simulink model "linearni_quad_trajektorie"  (R2020a)
settings: Solver=VariableStepAuto  StartTime=0.0  StopTime=smax/v  RelTol=1e-3
values from neighbouring files (symbols this model uses):
  a1 = 2    [overeniFunkcionality.m]    (also in sampleQnorm.m)
  a2 = 1.5    [overeniFunkcionality.m]    (also in sampleQnorm.m)
  a3 = 0.5    [overeniFunkcionality.m]    (also in sampleQnorm.m)
  r = a1-a2-a3    (= 0)    [overeniFunkcionality.m]    (also in sampleQnorm.m)
  R = a1+a2+a3    (= 4)    [overeniFunkcionality.m]    (also in sampleQnorm.m)
  s = surf(simulation.s_lin.signals.values,fiss,dQ)    [sampleQnorm.m]
  T_1_0 = [cos(theta10), -sin(theta10), 0, a1*cos(theta10) ... (first row only)    [overeniFunkcionality.m]    (also in sampleQnorm.m)
  T_2_1 = [cos(theta20), -sin(theta20), 0, a2*cos(theta20) ... (first row only)    [overeniFunkcionality.m]    (also in sampleQnorm.m)
  T_3_2 = [cos(theta30), -sin(theta30), 0, a3*cos(theta30) ... (first row only)    [overeniFunkcionality.m]    (also in sampleQnorm.m)
  v = 0.5    [overeniFunkcionality.m]    (also in sampleQnorm.m)
undefined symbols (not defined in the file or in its folder): X, Y, Z
libraries: sm_lib x84, nesl_utility x48
(part 3 of 3)

== system linearni_quad_trajektorie/Manipulator4/LINK 1 ==
  note: SUBSYSTEM RAMENE
  T_CG_1_0 : sm_lib/Frames and Transforms/Rigid Transform  TranslationMethod=Cartesian  TranslationStandardOffset=0  TranslationLengthUnit=m  TranslationStandardAxis=+Z  TranslationCartesianOffset=T_1_0(1:3,4)/2  TranslationROffset=0  TranslationROffsetUnits=m  TranslationZOffset=0  TranslationZOffsetUnits=m  TranslationThetaOffset=0  TranslationThetaOffsetUnits=deg  RotationMethod=RotationMatrix  RotationAngleUnits=deg  RotationStandardAxis=+Z  RotationAngle=0.0  RotationArbitraryAxis=[0 0 1]  FollAlignAxisA=+X  BaseAlignAxisA=+Y  FollAlignAxisB=+Y  BaseAlignAxisB=+Z  RotationSequenceAxes=FollowerAxes  RotationSequence=XYX  RotationSequenceAngles=[0 0 0]  RotationSequenceAnglesUnits=deg  RotationMatrix=T_1_0(1:3,1:3)
  Transform prvniho vuci nultymu = T_1_0 : sm_lib/Frames and Transforms/Rigid Transform  TranslationMethod=Cartesian  TranslationStandardOffset=0  TranslationLengthUnit=m  TranslationStandardAxis=+Z  TranslationCartesianOffset=T_1_0(1:3,4)  TranslationROffset=0  TranslationROffsetUnits=m  TranslationZOffset=0  TranslationZOffsetUnits=m  TranslationThetaOffset=0  TranslationThetaOffsetUnits=deg  RotationMethod=RotationMatrix  RotationAngleUnits=deg  RotationStandardAxis=+Z  RotationAngle=0.0  RotationArbitraryAxis=[0 0 1]  FollAlignAxisA=+X  BaseAlignAxisA=+Y  FollAlignAxisB=+Y  BaseAlignAxisB=+Z  RotationSequenceAxes=FollowerAxes  RotationSequence=XYX  RotationSequenceAngles=[0 0 0]  RotationSequenceAnglesUnits=deg  RotationMatrix=T_1_0(1:3,1:3)
  graficky objekt : sm_lib/Body Elements/Brick Solid  GraphicAmbientColor=[0.15 0.15 0.15 1.0]  BasedOnType=Density  BrickDimensions=[a1 0.05 0.05]  BrickDimensionUnits=m  CenterOfMass=[0 0 0]  CenterOfMassUnits=m  GraphicDiffuseColor=[0.5 0.5 0.5]  Density=1000  DensityUnits=kg/m^3  DoExposeReferenceFrame=on  GraphicEmissiveColor=[0.0 0.0 0.0 1.0]  ExportEntireGeometry=off  SerializedFrames=<Frames/>  MarkerShape=Sphere  MarkerSize=10  GraphicType=FromGeometry  InertiaType=CalculateFromGeometry  Mass=1  MassUnits=kg  MomentsOfInertia=[1 1 1]  MomentsOfInertiaUnits=kg*m^2  GraphicOpacity=1.0  ProductsOfInertia=[0 0 0]  ProductsOfInertiaUnits=kg*m^2  GraphicShininess=75  GraphicSpecularColor=[0.5 0.5 0.5 1.0]  GraphicVisPropType=SimpleVisualProperties
  CS_A : PMIOPort  Side=Left
  CS_B : PMIOPort  Port=2  Side=Right
  connections:
  Transform prvniho vuci nultymu = T_1_0/LConn1 -- CS_A/RConn1 -- T_CG_1_0/LConn1
  CS_B/RConn1 -- Transform prvniho vuci nultymu = T_1_0/RConn1
  graficky objekt/RConn1 -- T_CG_1_0/RConn1

== system linearni_quad_trajektorie/Manipulator4/LINK 2 ==
  note: SUBSYSTEM RAMENE
  T_CG_2_1 : sm_lib/Frames and Transforms/Rigid Transform  TranslationMethod=Cartesian  TranslationStandardOffset=0  TranslationLengthUnit=m  TranslationStandardAxis=+Z  TranslationCartesianOffset=T_2_1(1:3,4)/2  TranslationROffset=0  TranslationROffsetUnits=m  TranslationZOffset=0  TranslationZOffsetUnits=m  TranslationThetaOffset=0  TranslationThetaOffsetUnits=deg  RotationMethod=RotationMatrix  RotationAngleUnits=deg  RotationStandardAxis=+Z  RotationAngle=0.0  RotationArbitraryAxis=[0 0 1]  FollAlignAxisA=+X  BaseAlignAxisA=+Y  FollAlignAxisB=+Y  BaseAlignAxisB=+Z  RotationSequenceAxes=FollowerAxes  RotationSequence=XYX  RotationSequenceAngles=[0 0 0]  RotationSequenceAnglesUnits=deg  RotationMatrix=T_2_1(1:3,1:3)
  Transform druhyho vuci prvnimu = T_2_1 : sm_lib/Frames and Transforms/Rigid Transform  TranslationMethod=Cartesian  TranslationStandardOffset=0  TranslationLengthUnit=m  TranslationStandardAxis=+Z  TranslationCartesianOffset=T_2_1(1:3,4)  TranslationROffset=0  TranslationROffsetUnits=m  TranslationZOffset=0  TranslationZOffsetUnits=m  TranslationThetaOffset=0  TranslationThetaOffsetUnits=deg  RotationMethod=RotationMatrix  RotationAngleUnits=deg  RotationStandardAxis=+Z  RotationAngle=0.0  RotationArbitraryAxis=[0 0 1]  FollAlignAxisA=+X  BaseAlignAxisA=+Y  FollAlignAxisB=+Y  BaseAlignAxisB=+Z  RotationSequenceAxes=FollowerAxes  RotationSequence=XYX  RotationSequenceAngles=[0 0 0]  RotationSequenceAnglesUnits=deg  RotationMatrix=T_2_1(1:3,1:3)
  graficky objekt : sm_lib/Body Elements/Brick Solid  GraphicAmbientColor=[0.15 0.15 0.15 1.0]  BasedOnType=Density  BrickDimensions=[a2 0.05 0.05]  BrickDimensionUnits=m  CenterOfMass=[0 0 0]  CenterOfMassUnits=m  GraphicDiffuseColor=[0.5 0.5 0.5]  Density=1000  DensityUnits=kg/m^3  DoExposeReferenceFrame=on  GraphicEmissiveColor=[0.0 0.0 0.0 1.0]  ExportEntireGeometry=off  SerializedFrames=<Frames/>  MarkerShape=Sphere  MarkerSize=10  GraphicType=FromGeometry  InertiaType=CalculateFromGeometry  Mass=1  MassUnits=kg  MomentsOfInertia=[1 1 1]  MomentsOfInertiaUnits=kg*m^2  GraphicOpacity=1.0  ProductsOfInertia=[0 0 0]  ProductsOfInertiaUnits=kg*m^2  GraphicShininess=75  GraphicSpecularColor=[0.5 0.5 0.5 1.0]  GraphicVisPropType=SimpleVisualProperties
  CS_A : PMIOPort  Side=Left
  CS_B : PMIOPort  Port=2  Side=Right
  connections:
  T_CG_2_1/LConn1 -- Transform druhyho vuci prvnimu = T_2_1/LConn1 -- CS_A/RConn1
  CS_B/RConn1 -- Transform druhyho vuci prvnimu = T_2_1/RConn1
  graficky objekt/RConn1 -- T_CG_2_1/RConn1

== system linearni_quad_trajektorie/Manipulator4/LINK 3 ==
  note: SUBSYSTEM RAMENE
  T_CG_3_2 : sm_lib/Frames and Transforms/Rigid Transform  TranslationMethod=Cartesian  TranslationStandardOffset=0  TranslationLengthUnit=m  TranslationStandardAxis=+Z  TranslationCartesianOffset=T_3_2(1:3,4)/2  TranslationROffset=0  TranslationROffsetUnits=m  TranslationZOffset=0  TranslationZOffsetUnits=m  TranslationThetaOffset=0  TranslationThetaOffsetUnits=deg  RotationMethod=RotationMatrix  RotationAngleUnits=deg  RotationStandardAxis=+Z  RotationAngle=0.0  RotationArbitraryAxis=[0 0 1]  FollAlignAxisA=+X  BaseAlignAxisA=+Y  FollAlignAxisB=+Y  BaseAlignAxisB=+Z  RotationSequenceAxes=FollowerAxes  RotationSequence=XYX  RotationSequenceAngles=[0 0 0]  RotationSequenceAnglesUnits=deg  RotationMatrix=T_3_2(1:3,1:3)
  Transform tretiho vuci druhymu = T_3_2 : sm_lib/Frames and Transforms/Rigid Transform  TranslationMethod=Cartesian  TranslationStandardOffset=0  TranslationLengthUnit=m  TranslationStandardAxis=+Z  TranslationCartesianOffset=T_3_2(1:3,4)  TranslationROffset=0  TranslationROffsetUnits=m  TranslationZOffset=0  TranslationZOffsetUnits=m  TranslationThetaOffset=0  TranslationThetaOffsetUnits=deg  RotationMethod=RotationMatrix  RotationAngleUnits=deg  RotationStandardAxis=+Z  RotationAngle=0.0  RotationArbitraryAxis=[0 0 1]  FollAlignAxisA=+X  BaseAlignAxisA=+Y  FollAlignAxisB=+Y  BaseAlignAxisB=+Z  RotationSequenceAxes=FollowerAxes  RotationSequence=XYX  RotationSequenceAngles=[0 0 0]  RotationSequenceAnglesUnits=deg  RotationMatrix=T_3_2(1:3,1:3)
  graficky objekt : sm_lib/Body Elements/Brick Solid  GraphicAmbientColor=[0.15 0.15 0.15 1.0]  BasedOnType=Density  BrickDimensions=[a3 0.05 0.05]  BrickDimensionUnits=m  CenterOfMass=[0 0 0]  CenterOfMassUnits=m  GraphicDiffuseColor=[0.5 0.5 0.5]  Density=1000  DensityUnits=kg/m^3  DoExposeReferenceFrame=on  GraphicEmissiveColor=[0.0 0.0 0.0 1.0]  ExportEntireGeometry=off  SerializedFrames=<Frames/>  MarkerShape=Sphere  MarkerSize=10  GraphicType=FromGeometry  InertiaType=CalculateFromGeometry  Mass=1  MassUnits=kg  MomentsOfInertia=[1 1 1]  MomentsOfInertiaUnits=kg*m^2  GraphicOpacity=1.0  ProductsOfInertia=[0 0 0]  ProductsOfInertiaUnits=kg*m^2  GraphicShininess=75  GraphicSpecularColor=[0.5 0.5 0.5 1.0]  GraphicVisPropType=SimpleVisualProperties
  CS_A : PMIOPort  Side=Left
  CS_B : PMIOPort  Port=2  Side=Right
  connections:
  T_CG_3_2/LConn1 -- Transform tretiho vuci druhymu = T_3_2/LConn1 -- CS_A/RConn1
  CS_B/RConn1 -- Transform tretiho vuci druhymu = T_3_2/RConn1
  graficky objekt/RConn1 -- T_CG_3_2/RConn1

== matlab function linearni_quad_trajektorie/Linearni phi trajektorie1 ==
  data: s input; Xstar output size=3; v input; a input; dXstar output size=3; ddXstar output size=3
function [Xstar, dXstar, ddXstar] = MCSstar(s, v, a)

    A = [2 0.5]';
    B = [0 1]';
%     B = [1 1]';
    C = [2 2.5]';
%     sC = -A;

    r = 0.3;
    vmax = 1;
    
    fi_s = pi/2;
    fi_e = 0;
    
    if v > vmax
        v = vmax;
    else
        v = v;
    end
    nba = (A - B)/norm(A-B);
    nbc = (C-B)/norm(C-B);
    nbs = (nba+nbc)/norm(nba+nbc);
    K1 = (nba*nba'*nbs-nbs);
    l = r/(sqrt(K1'*K1));
    S = B+nbs*l;
    k = nba'*(A-S);
    Pa = A-nba*k;
    Pc = B + norm(Pa-B)*nbc;
    
%     
%     x_pab = A-k1.*nba
    Pb = B;

    helper = (Pa-S);
    fi_pa = atan2(helper(2),helper(1));
    dir = -1;
    deltafi = acos(((Pc-S)'*(Pa-S))/r^2);
    
    s1 = norm(Pa-A);
    s2 = norm(Pc-C);
    sk = r*deltafi;
    smax = s1+s2+sk;
    if s < s1
        k1 = s;
        dk1 = v;
        ddk1 = a;
        Xstar_tmp = A-k1*nba;
        dXstar_tmp = -dk1*nba;
        ddXstar_tmp = -ddk1*nba;
    elseif s1 <= s &&  s < s1+sk
        Phi = (s-s1)/r;
        dPhi = v/r;
        ddPhi = a/r;
        
        Xstar_tmp = r* [cos(fi_pa + dir*Phi); sin(fi_pa + dir*Phi)] + S;
        dXstar_tmp = r* [-sin(fi_pa + dir*Phi); cos(fi_pa + dir*Phi)]*dir*dPhi;
        ddXstar_tmp = r* [-cos(fi_pa + dir*Phi); -sin(fi_pa + dir*Phi)]*dPhi^2 + r* [-sin(fi_pa + dir*Phi); cos(fi_pa + dir*Phi)]*dir*ddPhi;
    elseif s1+sk < s && s < s1+sk+s2
        k2 = s-s1-sk;
        dk2 = v;
        ddk2 = a;
        
        Xstar_tmp = Pc + k2*nbc;
        dXstar_tmp = dk2*nbc;
        ddXstar_tmp = ddk2*nbc;
    else
%         display('ERROR V TRAJEKTORII')
        Xstar_tmp = C;
        dXstar_tmp = zeros(2,1);
        ddXstar_tmp = zeros(2,1);
    end
    
    
    fi = fi_s - fi_s/smax*s;
    dfi = -fi_s/(smax/v);
    ddfi = 0;

    
    Xstar = [Xstar_tmp; fi];
    dXstar = [dXstar_tmp; dfi];
    ddXstar = [ddXstar_tmp; ddfi];
    
end

== matlab function linearni_quad_trajektorie/MATLAB Function2 ==
  data: x input; y input; phi input; dx input; dy input; dphi input; ddx input; ddy input; ddphi input; a1 parameter; a2 parameter; a3 parameter; theta1 output size=1; theta2 output size=1; theta3 output size=1; theta1_dot output size=1; theta2_dot output size=1; theta3_dot output size=1; theta1_dot_dot output size=1; theta2_dot_dot output size=1; theta3_dot_dot output size=1
function [theta1, theta2, theta3,theta1_dot,theta2_dot,theta3_dot,theta1_dot_dot,theta2_dot_dot,theta3_dot_dot] = IOKU( x, y, phi, dx, dy, dphi, ddx, ddy, ddphi, a1, a2, a3)

% theta2
cosQ2 = ((x - a3*cos(phi))^2 + (y - a3*sin(phi))^2 - a1^2 - a2^2)/(2 * a1 * a2);
sinQ2 = -abs(sqrt(abs(1 - cosQ2^2)));
theta2 = atan2(sinQ2, cosQ2);

% theta1
A = [-a2 * sin(theta2), a2 * cos(theta2) + a1; a2 * cos(theta2) + a1, a2 * sin(theta2)];
B = [x - a3*cos(phi); y - a3*sin(phi)];
X = A\B;
theta1 = atan2(X(1), X(2));

% theta3
theta3 = phi - theta1 - theta2;

% uhlova rychlost
JQ = [-a3 * sin(theta1 + theta2 + theta3) - a2 * sin(theta1 + theta2) - a1 * sin(theta1), -a3 * sin(theta1 + theta2 + theta3) - a2 * sin(theta1 + theta2), -a3 * sin(theta1 + theta2 + theta3);...
       a3 * cos(theta1 + theta2 + theta3) + a2 * cos(theta1 + theta2) + a1 * cos(theta1), a3 * cos(theta1 + theta2 + theta3) + a2 * cos(theta1 + theta2), a3 * cos(theta1 + theta2 + theta3);...
       1, 1, 1];
dX = [dx; dy; dphi];
dQ = JQ^(-1) * dX;
theta1_dot = dQ(1);
theta2_dot = dQ(2);
theta3_dot = dQ(3);

% uhlove zrychleni
dJQ = [-a3*cos(theta1+theta2+theta3)*(theta1_dot+theta2_dot+theta3_dot) - a2*cos(theta1+theta2)*(theta1_dot+theta2_dot) - a1*cos(theta1)*theta1_dot, -a3*cos(theta1+theta2+theta3)*(theta1_dot+theta2_dot+theta3_dot) - a2*cos(theta1+theta2)*(theta1_dot+theta2_dot), -a3*cos(theta1+theta2+theta3)*(theta1_dot+theta2_dot+theta3_dot);...
    -a3*sin(theta1+theta2+theta3)*(theta1_dot+theta2_dot+theta3_dot) - a2*sin(theta1+theta2)*(theta1_dot+theta2_dot) - a1*sin(theta1)*theta1_dot, -a3*sin(theta1+theta2+theta3)*(theta1_dot+theta2_dot+theta3_dot) - a2*sin(theta1+theta2)*(theta1_dot+theta2_dot), -a3*sin(theta1+theta2+theta3)*(theta1_dot+theta2_dot+theta3_dot);...
    0, 0, 0];
ddX = [ddx; ddy; ddphi];
ddQ = JQ^(-1) * (ddX - dJQ * dQ);
theta1_dot_dot = ddQ(1);
theta2_dot_dot = ddQ(2);
theta3_dot_dot = ddQ(3);


end

== matlab function linearni_quad_trajektorie/norm calculation2 ==
  data: u1 input; normQ output size=1; u2 input; u3 input
function normQ   = make_norm(u1,u2,u3)
    normQ = norm([u1,u2,u3]);


end

== matlab function linearni_quad_trajektorie/MATLAB Function17 ==
  data: x input; y input; phi input; dx input; dy input; dphi input; ddx input; ddy input; ddphi input; a1 parameter; a2 parameter; a3 parameter; theta1 output size=1; theta2 output size=1; theta3 output size=1; theta1_dot output size=1; theta2_dot output size=1; theta3_dot output size=1; theta1_dot_dot output size=1; theta2_dot_dot output size=1; theta3_dot_dot output size=1
function [theta1, theta2, theta3,theta1_dot,theta2_dot,theta3_dot,theta1_dot_dot,theta2_dot_dot,theta3_dot_dot] = IOKU( x, y, phi, dx, dy, dphi, ddx, ddy, ddphi, a1, a2, a3)

% theta2
cosQ2 = ((x - a3*cos(phi))^2 + (y - a3*sin(phi))^2 - a1^2 - a2^2)/(2 * a1 * a2);
sinQ2 = -abs(sqrt(abs(1 - cosQ2^2)));
theta2 = atan2(sinQ2, cosQ2);

% theta1
A = [-a2 * sin(theta2), a2 * cos(theta2) + a1; a2 * cos(theta2) + a1, a2 * sin(theta2)];
B = [x - a3*cos(phi); y - a3*sin(phi)];
X = A\B;
theta1 = atan2(X(1), X(2));

% theta3
theta3 = phi - theta1 - theta2;

% uhlova rychlost
JQ = [-a3 * sin(theta1 + theta2 + theta3) - a2 * sin(theta1 + theta2) - a1 * sin(theta1), -a3 * sin(theta1 + theta2 + theta3) - a2 * sin(theta1 + theta2), -a3 * sin(theta1 + theta2 + theta3);...
       a3 * cos(theta1 + theta2 + theta3) + a2 * cos(theta1 + theta2) + a1 * cos(theta1), a3 * cos(theta1 + theta2 + theta3) + a2 * cos(theta1 + theta2), a3 * cos(theta1 + theta2 + theta3);...
       1, 1, 1];
dX = [dx; dy; dphi];
dQ = JQ^(-1) * dX;
theta1_dot = dQ(1);
theta2_dot = dQ(2);
theta3_dot = dQ(3);

% uhlove zrychleni
dJQ = [-a3*cos(theta1+theta2+theta3)*(theta1_dot+theta2_dot+theta3_dot) - a2*cos(theta1+theta2)*(theta1_dot+theta2_dot) - a1*cos(theta1)*theta1_dot, -a3*cos(theta1+theta2+theta3)*(theta1_dot+theta2_dot+theta3_dot) - a2*cos(theta1+theta2)*(theta1_dot+theta2_dot), -a3*cos(theta1+theta2+theta3)*(theta1_dot+theta2_dot+theta3_dot);...
    -a3*sin(theta1+theta2+theta3)*(theta1_dot+theta2_dot+theta3_dot) - a2*sin(theta1+theta2)*(theta1_dot+theta2_dot) - a1*sin(theta1)*theta1_dot, -a3*sin(theta1+theta2+theta3)*(theta1_dot+theta2_dot+theta3_dot) - a2*sin(theta1+theta2)*(theta1_dot+theta2_dot), -a3*sin(theta1+theta2+theta3)*(theta1_dot+theta2_dot+theta3_dot);...
    0, 0, 0];
ddX = [ddx; ddy; ddphi];
ddQ = JQ^(-1) * (ddX - dJQ * dQ);
theta1_dot_dot = ddQ(1);
theta2_dot_dot = ddQ(2);
theta3_dot_dot = ddQ(3);


end

== matlab function linearni_quad_trajektorie/Linearni phi trajektorie ==
  data: s input; Xstar output size=3; v input; a input; dXstar output size=3; ddXstar output size=3
function [Xstar, dXstar, ddXstar] = MCSstar(s, v, a)

    A = [2 0.5]';
    B = [0 1]';
%     B = [1 1]';
    C = [2 2.5]';
%     sC = -A;

    r = 0.3;
    vmax = 1;
    
    fi_s = pi/2;
    fi_e = 0;
    
    if v > vmax
        v = vmax;
    else
        v = v;
    end
    nba = (A - B)/norm(A-B);
    nbc = (C-B)/norm(C-B);
    nbs = (nba+nbc)/norm(nba+nbc);
    K1 = (nba*nba'*nbs-nbs);
    l = r/(sqrt(K1'*K1));
    S = B+nbs*l;
    k = nba'*(A-S);
    Pa = A-nba*k;
    Pc = B + norm(Pa-B)*nbc;
    
%     
%     x_pab = A-k1.*nba
    Pb = B;

    helper = (Pa-S);
    fi_pa = atan2(helper(2),helper(1));
    dir = -1;
    deltafi = acos(((Pc-S)'*(Pa-S))/r^2);
    
    s1 = norm(Pa-A);
    s2 = norm(Pc-C);
    sk = r*deltafi;
    smax = s1+s2+sk;
    if s < s1
        k1 = s;
        dk1 = v;
        ddk1 = a;
        Xstar_tmp = A-k1*nba;
        dXstar_tmp = -dk1*nba;
        ddXstar_tmp = -ddk1*nba;
    elseif s1 <= s &&  s < s1+sk
        Phi = (s-s1)/r;
        dPhi = v/r;
        ddPhi = a/r;
        
        Xstar_tmp = r* [cos(fi_pa + dir*Phi); sin(fi_pa + dir*Phi)] + S;
        dXstar_tmp = r* [-sin(fi_pa + dir*Phi); cos(fi_pa + dir*Phi)]*dir*dPhi;
        ddXstar_tmp = r* [-cos(fi_pa + dir*Phi); -sin(fi_pa + dir*Phi)]*dPhi^2 + r* [-sin(fi_pa + dir*Phi); cos(fi_pa + dir*Phi)]*dir*ddPhi;
    elseif s1+sk < s && s < s1+sk+s2
        k2 = s-s1-sk;
        dk2 = v;
        ddk2 = a;
        
        Xstar_tmp = Pc + k2*nbc;
        dXstar_tmp = dk2*nbc;
        ddXstar_tmp = ddk2*nbc;
    else
%         display('ERROR V TRAJEKTORII')
        Xstar_tmp = C;
        dXstar_tmp = zeros(2,1);
        ddXstar_tmp = zeros(2,1);
    end
    
    
    fi = fi_s - fi_s/smax*s;
    dfi = -fi_s/(smax/v);
    ddfi = 0;

    
    Xstar = [Xstar_tmp; fi];
    dXstar = [dXstar_tmp; dfi];
    ddXstar = [ddXstar_tmp; ddfi];
    
end

== matlab function linearni_quad_trajektorie/konstantni phi ==
  data: s input; Xstar output size=3; v input; a input; dXstar output size=3; ddXstar output size=3; fi_sample parameter
function [Xstar, dXstar, ddXstar] = MCSstar(s, v, a, fi_sample)

    A = [2 0.5]';
    B = [0 1]';
%     B = [1 1]';
    C = [2 2.5]';
%     sC = -A;

    r = 0.3;
    vmax = 1;
    
    fi_s = pi/2;
    fi_e = 0;
    
    if v > vmax
        v = vmax;
    else
        v = v;
    end
    nba = (A - B)/norm(A-B);
    nbc = (C-B)/norm(C-B);
    nbs = (nba+nbc)/norm(nba+nbc);
    K1 = (nba*nba'*nbs-nbs);
    l = r/(sqrt(K1'*K1));
    S = B+nbs*l;
    k = nba'*(A-S);
    Pa = A-nba*k;
    Pc = B + norm(Pa-B)*nbc;
    
%     
%     x_pab = A-k1.*nba
    Pb = B;

    helper = (Pa-S);
    fi_pa = atan2(helper(2),helper(1));
    dir = -1;
    deltafi = acos(((Pc-S)'*(Pa-S))/r^2);
    
    s1 = norm(Pa-A);
    s2 = norm(Pc-C);
    sk = r*deltafi;
    smax = s1+s2+sk;
    if s < s1
        k1 = s;
        dk1 = v;
        ddk1 = a;
        Xstar_tmp = A-k1*nba;
        dXstar_tmp = -dk1*nba;
        ddXstar_tmp = -ddk1*nba;
    elseif s1 <= s &&  s < s1+sk
        Phi = (s-s1)/r;
        dPhi = v/r;
        ddPhi = a/r;
        
        Xstar_tmp = r* [cos(fi_pa + dir*Phi); sin(fi_pa + dir*Phi)] + S;
        dXstar_tmp = r* [-sin(fi_pa + dir*Phi); cos(fi_pa + dir*Phi)]*dir*dPhi;
        ddXstar_tmp = r* [-cos(fi_pa + dir*Phi); -sin(fi_pa + dir*Phi)]*dPhi^2 + r* [-sin(fi_pa + dir*Phi); cos(fi_pa + dir*Phi)]*dir*ddPhi;
    elseif s1+sk < s && s < s1+sk+s2
        k2 = s-s1-sk;
        dk2 = v;
        ddk2 = a;
        
        Xstar_tmp = Pc + k2*nbc;
        dXstar_tmp = dk2*nbc;
        ddXstar_tmp = ddk2*nbc;
    else
%         display('ERROR V TRAJEKTORII')
        Xstar_tmp = C;
        dXstar_tmp = zeros(2,1);
        ddXstar_tmp = zeros(2,1);
    end
    
    fi = fi_sample;
    dfi = 0;
    ddfi = 0;

    Xstar = [Xstar_tmp; fi];
    dXstar = [dXstar_tmp; dfi];
    ddXstar = [ddXstar_tmp; ddfi];
    
   
%     
%     k1 = linspace(0,norm(A-Pa),100)
% 
% 
%     
%     fi = linspace(0,deltafi,100)
%     x_rot = [r*cos(fi_pa+dir*fi);
%              r*sin(fi_pa+dir*fi)]+S
% 
%     k2 = linspace(0,norm(Pc-C),100)
%     x_pbc = Pc + k2.*nbc
% 
% 
% 
%     smax = s1+s2+sk
%     Tmax = smax/vmax
% 
%     T = 100
%     t = linspace(0,Tmax,T)
%     t1 = linspace(0,s1/vmax,T)
%     tk = linspace(s1/vmax,sk/vmax,T)
%     t2 = linspace(sk/vmax,s2/vmax,T)
%     % s = linspace(0,smax,smax/Tmax*10)
%     s = vmax*t
% 
% 
%     k1 = 0+vmax*t
% 
%     k1 = linspace(0,s1,s1/Tmax*T)
%     fi = linspace(0,(sk)/r,(sk)/Tmax*T)
%     k2 = linspace(0,s2,s2/Tmax*T)
% 
%     
%     Xk = [r*cos(fi_pa+dir*fi);r*sin(fi_pa+dir*fi)]+S
%     X2 = Pc+k2.*nbc


end

== matlab function linearni_quad_trajektorie/MATLAB Function1 ==
  data: x input; y input; phi input; dx input; dy input; dphi input; ddx input; ddy input; ddphi input; a1 parameter; a2 parameter; a3 parameter; theta1 output size=1; theta2 output size=1; theta3 output size=1; theta1_dot output size=1; theta2_dot output size=1; theta3_dot output size=1; theta1_dot_dot output size=1; theta2_dot_dot output size=1; theta3_dot_dot output size=1
function [theta1, theta2, theta3,theta1_dot,theta2_dot,theta3_dot,theta1_dot_dot,theta2_dot_dot,theta3_dot_dot] = IOKU( x, y, phi, dx, dy, dphi, ddx, ddy, ddphi, a1, a2, a3)

% theta2
cosQ2 = ((x - a3*cos(phi))^2 + (y - a3*sin(phi))^2 - a1^2 - a2^2)/(2 * a1 * a2);
sinQ2 = -abs(sqrt(abs(1 - cosQ2^2)));
theta2 = atan2(sinQ2, cosQ2);

% theta1
A = [-a2 * sin(theta2), a2 * cos(theta2) + a1; a2 * cos(theta2) + a1, a2 * sin(theta2)];
B = [x - a3*cos(phi); y - a3*sin(phi)];
X = A\B;
theta1 = atan2(X(1), X(2));

% theta3
theta3 = phi - theta1 - theta2;

% uhlova rychlost
JQ = [-a3 * sin(theta1 + theta2 + theta3) - a2 * sin(theta1 + theta2) - a1 * sin(theta1), -a3 * sin(theta1 + theta2 + theta3) - a2 * sin(theta1 + theta2), -a3 * sin(theta1 + theta2 + theta3);...
       a3 * cos(theta1 + theta2 + theta3) + a2 * cos(theta1 + theta2) + a1 * cos(theta1), a3 * cos(theta1 + theta2 + theta3) + a2 * cos(theta1 + theta2), a3 * cos(theta1 + theta2 + theta3);...
       1, 1, 1];
dX = [dx; dy; dphi];
dQ = JQ^(-1) * dX;
theta1_dot = dQ(1);
theta2_dot = dQ(2);
theta3_dot = dQ(3);

% uhlove zrychleni
dJQ = [-a3*cos(theta1+theta2+theta3)*(theta1_dot+theta2_dot+theta3_dot) - a2*cos(theta1+theta2)*(theta1_dot+theta2_dot) - a1*cos(theta1)*theta1_dot, -a3*cos(theta1+theta2+theta3)*(theta1_dot+theta2_dot+theta3_dot) - a2*cos(theta1+theta2)*(theta1_dot+theta2_dot), -a3*cos(theta1+theta2+theta3)*(theta1_dot+theta2_dot+theta3_dot);...
    -a3*sin(theta1+theta2+theta3)*(theta1_dot+theta2_dot+theta3_dot) - a2*sin(theta1+theta2)*(theta1_dot+theta2_dot) - a1*sin(theta1)*theta1_dot, -a3*sin(theta1+theta2+theta3)*(theta1_dot+theta2_dot+theta3_dot) - a2*sin(theta1+theta2)*(theta1_dot+theta2_dot), -a3*sin(theta1+theta2+theta3)*(theta1_dot+theta2_dot+theta3_dot);...
    0, 0, 0];
ddX = [ddx; ddy; ddphi];
ddQ = JQ^(-1) * (ddX - dJQ * dQ);
theta1_dot_dot = ddQ(1);
theta2_dot_dot = ddQ(2);
theta3_dot_dot = ddQ(3);


end

== matlab function linearni_quad_trajektorie/norm calculation ==
  data: u1 input; normQ output size=1; u2 input; u3 input
function normQ   = make_norm(u1,u2,u3)
    normQ = norm([u1,u2,u3]);


end

== matlab function linearni_quad_trajektorie/norm calculation1 ==
  data: u1 input; normQ output size=1; u2 input; u3 input
function normQ   = make_norm(u1,u2,u3)
    normQ = norm([u1,u2,u3]);


end

== matlab function linearni_quad_trajektorie/Linearni phi trajektorie s zastavkou ==
  data: s input; Xstar output size=3; v input; a input; dXstar output size=3; ddXstar output size=3
function [Xstar, dXstar, ddXstar] = MCSstar(s, v, a)

    A = [2 0.5]';
    B = [0 1]';
%     B = [1 1]';
    C = [2 2.5]';
%     sC = -A;

    r = 0.3;
    vmax = 1;
    
    fi_s = pi/2;
    fi_e = 0;
    
    if v > vmax
        v = vmax;
    else
        v = v;
    end
    nba = (A - B)/norm(A-B);
    nbc = (C-B)/norm(C-B);
    nbs = (nba+nbc)/norm(nba+nbc);
    K1 = (nba*nba'*nbs-nbs);
    l = r/(sqrt(K1'*K1));
    S = B+nbs*l;
    k = nba'*(A-S);
    Pa = A-nba*k;
    Pc = B + norm(Pa-B)*nbc;
    
%     
%     x_pab = A-k1.*nba
    Pb = B;

    helper = (Pa-S);
    fi_pa = atan2(helper(2),helper(1));
    dir = -1;
    deltafi = acos(((Pc-S)'*(Pa-S))/r^2);
    
    s1 = norm(Pa-A);
    s2 = norm(Pc-C);
    sk = r*deltafi;
    smax = s1+s2+sk;
    if s < s1
        k1 = s;
        dk1 = v;
        ddk1 = a;
        Xstar_tmp = A-k1*nba;
        dXstar_tmp = -dk1*nba;
        ddXstar_tmp = -ddk1*nba;
    elseif s1 <= s &&  s < s1+sk
        Phi = (s-s1)/r;
        dPhi = v/r;
        ddPhi = a/r;
        
        Xstar_tmp = r* [cos(fi_pa + dir*Phi); sin(fi_pa + dir*Phi)] + S;
        dXstar_tmp = r* [-sin(fi_pa + dir*Phi); cos(fi_pa + dir*Phi)]*dir*dPhi;
        ddXstar_tmp = r* [-cos(fi_pa + dir*Phi); -sin(fi_pa + dir*Phi)]*dPhi^2 + r* [-sin(fi_pa + dir*Phi); cos(fi_pa + dir*Phi)]*dir*ddPhi;
    elseif s1+sk < s && s < s1+sk+s2
        k2 = s-s1-sk;
        dk2 = v;
        ddk2 = a;
        
        Xstar_tmp = Pc + k2*nbc;
        dXstar_tmp = dk2*nbc;
        ddXstar_tmp = ddk2*nbc;
    else
%         display('ERROR V TRAJEKTORII')
        Xstar_tmp = C;
        dXstar_tmp = zeros(2,1);
        ddXstar_tmp = zeros(2,1);
    end
    
    
    fi = fi_s - fi_s/smax*s;
    dfi = -fi_s/(smax/v);
    ddfi = 0;
    if 1 < s && s <2.5
        fi = fi_s - fi_s/smax*1;
        dfi = 0;
        ddfi = 0;
    elseif s > 2.5
        fi = fi_s - fi_s/smax*(s - (2.5-1));
        dfi = -fi_s/(smax/v);
        ddfi = 0;
    end
    
    Xstar = [Xstar_tmp; fi];
    dXstar = [dXstar_tmp; dfi];
    ddXstar = [ddXstar_tmp; ddfi];
    
end

== matlab function linearni_quad_trajektorie/Kvadraticka phi trajektorie ==
  data: s input; Xstar output size=3; v input; a input; dXstar output size=3; ddXstar output size=3
function [Xstar, dXstar, ddXstar] = MCSstar(s, v, a)

    A = [2 0.5]';
    B = [0 1]';
%     B = [1 1]';
    C = [2 2.5]';
%     sC = -A;

    r = 0.3;
    vmax = 1;
    
    fi_s = pi/2;
    fi_e = 0;
    
    if v > vmax
        v = vmax;
    else
        v = v;
    end
    nba = (A - B)/norm(A-B);
    nbc = (C-B)/norm(C-B);
    nbs = (nba+nbc)/norm(nba+nbc);
    K1 = (nba*nba'*nbs-nbs);
    l = r/(sqrt(K1'*K1));
    S = B+nbs*l;
    k = nba'*(A-S);
    Pa = A-nba*k;
    Pc = B + norm(Pa-B)*nbc;
    
%     
%     x_pab = A-k1.*nba
    Pb = B;

    helper = (Pa-S);
    fi_pa = atan2(helper(2),helper(1));
    dir = -1;
    deltafi = acos(((Pc-S)'*(Pa-S))/r^2);
    
    s1 = norm(Pa-A);
    s2 = norm(Pc-C);
    sk = r*deltafi;
    smax = s1+s2+sk;
    if s < s1
        k1 = s;
        dk1 = v;
        ddk1 = a;
        Xstar_tmp = A-k1*nba;
        dXstar_tmp = -dk1*nba;
        ddXstar_tmp = -ddk1*nba;
    elseif s1 <= s &&  s < s1+sk
        Phi = (s-s1)/r;
        dPhi = v/r;
        ddPhi = a/r;
        
        Xstar_tmp = r* [cos(fi_pa + dir*Phi); sin(fi_pa + dir*Phi)] + S;
        dXstar_tmp = r* [-sin(fi_pa + dir*Phi); cos(fi_pa + dir*Phi)]*dir*dPhi;
        ddXstar_tmp = r* [-cos(fi_pa + dir*Phi); -sin(fi_pa + dir*Phi)]*dPhi^2 + r* [-sin(fi_pa + dir*Phi); cos(fi_pa + dir*Phi)]*dir*ddPhi;
    elseif s1+sk < s && s < s1+sk+s2
        k2 = s-s1-sk;
        dk2 = v;
        ddk2 = a;
        
        Xstar_tmp = Pc + k2*nbc;
        dXstar_tmp = dk2*nbc;
        ddXstar_tmp = ddk2*nbc;
    else
%         display('ERROR V TRAJEKTORII')
        Xstar_tmp = C;
        dXstar_tmp = zeros(2,1);
        ddXstar_tmp = zeros(2,1);
    end
    
    %%

    
    xfit = [0 1.5 smax];
    yfit = [pi/2 -0 0];
    p = polyfit(xfit, yfit, 2);
    
    fi = p(1)*s^2 + p(2)*s + p(3);
    dfi = (2*p(1) + p(2))*v;
    ddfi = 0;

    
    Xstar = [Xstar_tmp; fi];
    dXstar = [dXstar_tmp; dfi];
    ddXstar = [ddXstar_tmp; ddfi];
    
end
